simulink model "task4_lab9"  (R2021a)
settings: Solver=VariableStepAuto  StartTime=0.0  StopTime=10.0  RelTol=1e-3
settings Model: Creator=reemb  LastModifiedBy=reemb

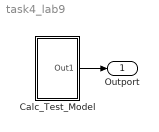
== system task4_lab9 ==
  Calc_Test_Model : Subsystem  TreatAsAtomicUnit=on  RTWFcnName=calc_functions
      settings: RTWFcnNameOpts=User specified  RTWFileNameOpts=Use function name
  Outport : Outport
  wires:
  Calc_Test_Model/1(Out1) -> Outport/1

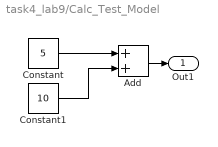
== system task4_lab9/Calc_Test_Model ==
  Add : Sum
  Constant : Constant  Value=5
  Constant1 : Constant  Value=10
  Out1 : Outport
  wires:
  Constant1/1 -> Add/2
  Constant/1 -> Add/1
  Add/1 -> Out1/1
